simulink model "stage_one"  (R2021b)
settings: Solver=VariableStepAuto  StartTime=0.0  StopTime=0.2  FixedStep=1e3  RelTol=1e-8
libraries: spsTriangleGeneratorLib x3
settings Model: Creator=Selected  LastModifiedBy=Selected
settings SolverCC: ShapePreserveControl=EnableAll

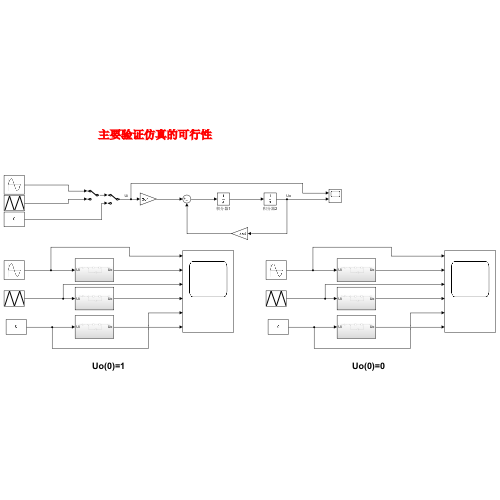
[thumbnail: Simulink's stored preview of the top-level diagram]
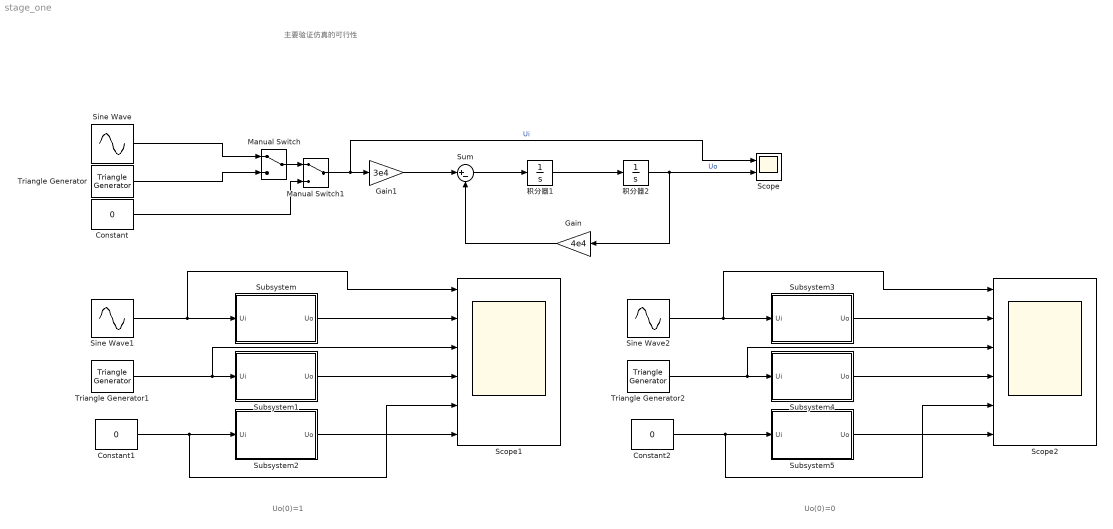
== system stage_one ==
  note: Uo(0)=0
  note: 主要验证仿真的可行性
  note: Uo(0)=1
  Constant : Constant  Value=0
  Constant1 : Constant  Value=0
  Constant2 : Constant  Value=0
  Gain : Gain  Gain=4e4
  Gain1 : Gain  Gain=3e4
  Manual Switch : ManualSwitch
  Manual Switch1 : ManualSwitch
  Scope : Scope  NumInputPorts=2
  Scope1 : Scope  NumInputPorts=6
  Scope2 : Scope  NumInputPorts=6
  Sine Wave : Sin  Amplitude=2  Frequency=600  SampleTime=0
  Sine Wave1 : Sin  Amplitude=2  Frequency=600  SampleTime=0
  Sine Wave2 : Sin  Amplitude=2  Frequency=600  SampleTime=0
  Subsystem : Subsystem
  Subsystem1 : Subsystem
  Subsystem2 : Subsystem
  Subsystem3 : Subsystem
  Subsystem4 : Subsystem
  Subsystem5 : Subsystem
  Sum : Sum  Inputs=|+-
  Triangle Generator : spsTriangleGeneratorLib/Triangle Generator  Freq=600/2/pi  Phase=0  Ts=0
  Triangle Generator1 : spsTriangleGeneratorLib/Triangle Generator  Freq=600/2/pi  Phase=0  Ts=0
  Triangle Generator2 : spsTriangleGeneratorLib/Triangle Generator  Freq=600/2/pi  Phase=0  Ts=0
  积分器1 : Integrator
  积分器2 : Integrator  InitialCondition=1
  wires:
  积分器1/1 -> 积分器2/1
  积分器2/1 -> Gain/1, Scope/2  "Uo"
  Gain/1 -> Sum/2
  Sum/1 -> 积分器1/1
  Gain1/1 -> Sum/1
  Manual Switch/1 -> Manual Switch1/1
  Sine Wave/1 -> Manual Switch/1
  Manual Switch1/1 -> Scope/1, Gain1/1  "Ui"
  Constant/1 -> Manual Switch1/2
  Triangle Generator/1 -> Manual Switch/2
  Sine Wave1/1 -> Scope1/1, Subsystem/1(Ui)
  Subsystem/1(Uo) -> Scope1/2
  Triangle Generator1/1 -> Subsystem1/1(Ui), Scope1/3
  Constant1/1 -> Scope1/5, Subsystem2/1(Ui)
  Subsystem1/1(Uo) -> Scope1/4
  Subsystem2/1(Uo) -> Scope1/6
  Subsystem5/1(Uo) -> Scope2/6
  Subsystem3/1(Uo) -> Scope2/2
  Triangle Generator2/1 -> Subsystem4/1(Ui), Scope2/3
  Subsystem4/1(Uo) -> Scope2/4
  Constant2/1 -> Scope2/5, Subsystem5/1(Ui)
  Sine Wave2/1 -> Scope2/1, Subsystem3/1(Ui)

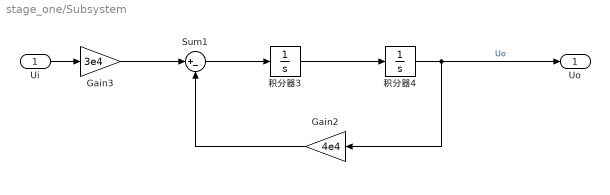
== system stage_one/Subsystem ==
  Ui : Inport
  Gain2 : Gain  Gain=4e4
  Gain3 : Gain  Gain=3e4
  Sum1 : Sum  Inputs=|+-
  积分器3 : Integrator
  积分器4 : Integrator  InitialCondition=1
  Uo : Outport
  wires:
  积分器4/1 -> Uo/1, Gain2/1  "Uo"
  积分器3/1 -> 积分器4/1
  Gain3/1 -> Sum1/1
  Gain2/1 -> Sum1/2
  Sum1/1 -> 积分器3/1
  Ui/1 -> Gain3/1

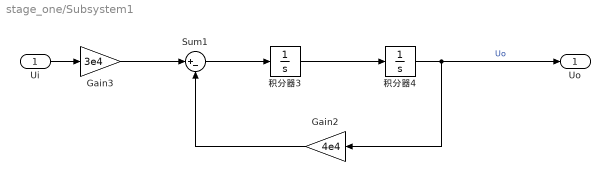
== system stage_one/Subsystem1 ==
  Ui : Inport
  Gain2 : Gain  Gain=4e4
  Gain3 : Gain  Gain=3e4
  Sum1 : Sum  Inputs=|+-
  积分器3 : Integrator
  积分器4 : Integrator  InitialCondition=1
  Uo : Outport
  wires:
  积分器4/1 -> Uo/1, Gain2/1  "Uo"
  积分器3/1 -> 积分器4/1
  Gain3/1 -> Sum1/1
  Gain2/1 -> Sum1/2
  Sum1/1 -> 积分器3/1
  Ui/1 -> Gain3/1

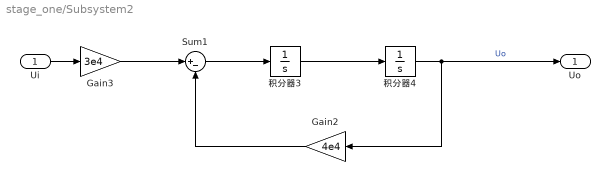
== system stage_one/Subsystem2 ==
  Ui : Inport
  Gain2 : Gain  Gain=4e4
  Gain3 : Gain  Gain=3e4
  Sum1 : Sum  Inputs=|+-
  积分器3 : Integrator
  积分器4 : Integrator  InitialCondition=1
  Uo : Outport
  wires:
  积分器4/1 -> Uo/1, Gain2/1  "Uo"
  积分器3/1 -> 积分器4/1
  Gain3/1 -> Sum1/1
  Gain2/1 -> Sum1/2
  Sum1/1 -> 积分器3/1
  Ui/1 -> Gain3/1

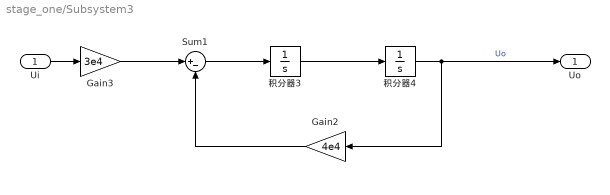
== system stage_one/Subsystem3 ==
  Ui : Inport
  Gain2 : Gain  Gain=4e4
  Gain3 : Gain  Gain=3e4
  Sum1 : Sum  Inputs=|+-
  积分器3 : Integrator
  积分器4 : Integrator
  Uo : Outport
  wires:
  积分器4/1 -> Uo/1, Gain2/1  "Uo"
  积分器3/1 -> 积分器4/1
  Gain3/1 -> Sum1/1
  Gain2/1 -> Sum1/2
  Sum1/1 -> 积分器3/1
  Ui/1 -> Gain3/1

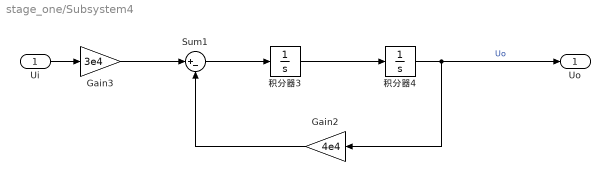
== system stage_one/Subsystem4 ==
  Ui : Inport
  Gain2 : Gain  Gain=4e4
  Gain3 : Gain  Gain=3e4
  Sum1 : Sum  Inputs=|+-
  积分器3 : Integrator
  积分器4 : Integrator
  Uo : Outport
  wires:
  积分器4/1 -> Uo/1, Gain2/1  "Uo"
  积分器3/1 -> 积分器4/1
  Gain3/1 -> Sum1/1
  Gain2/1 -> Sum1/2
  Sum1/1 -> 积分器3/1
  Ui/1 -> Gain3/1

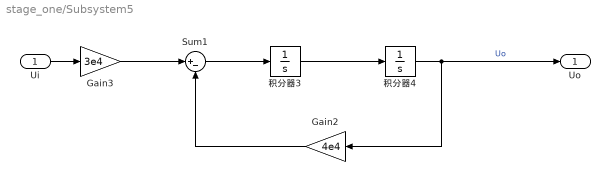
== system stage_one/Subsystem5 ==
  Ui : Inport
  Gain2 : Gain  Gain=4e4
  Gain3 : Gain  Gain=3e4
  Sum1 : Sum  Inputs=|+-
  积分器3 : Integrator
  积分器4 : Integrator
  Uo : Outport
  wires:
  积分器4/1 -> Uo/1, Gain2/1  "Uo"
  积分器3/1 -> 积分器4/1
  Gain3/1 -> Sum1/1
  Gain2/1 -> Sum1/2
  Sum1/1 -> 积分器3/1
  Ui/1 -> Gain3/1
